simulink subsystem "Rocket_Motor"  (R2020b)
settings: Solver=VariableStepAuto  StartTime=0.0  StopTime=10.0  RelTol=1e-3
undefined symbols (not defined in the file): LocalRestrictions
libraries: fl_lib x27, nesl_utility x18
settings Model: Creator=Edward  LastModifiedBy=Rafal

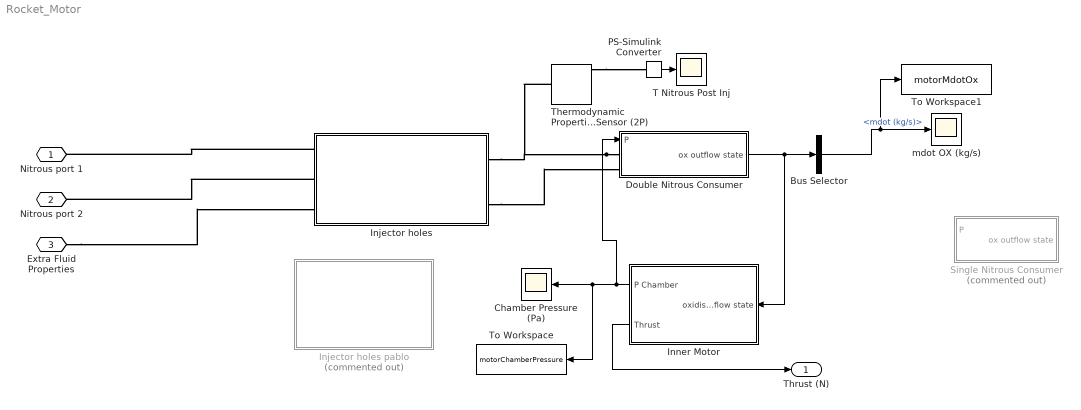
== system Rocket_Motor ==
  Bus Selector : BusSelector  OutputSignals=mdot (kg/s)
  Chamber Pressure (Pa) : Scope
  Double Nitrous Consumer : Subsystem
  Injector holes : Subsystem  Variant=on  VariantControlMode=label  VariantControl=Choice  LabelModeActiveChoice=Omega Modified
  Injector holes pablo : Subsystem  Commented=on
  Inner Motor : Subsystem
      mask Display: image('$imagefile'); % Use "Edit Image" on toolstrip to change.
  PS-Simulink Converter : nesl_utility/PS-Simulink Converter  PhysicalDomain=network_engine_domain  SubClassName=ps_output  LeftPortType=input  RightPortType=output  PseudoPeriodic=off  Frequencies=[]  Unit=inherit  AffineConversion=off
  Single Nitrous Consumer : Subsystem  Commented=on
  T Nitrous Post Inj : Scope
  Thermodynamic Properties Sensor (2P) : fl_lib/Two-Phase Fluid/Sensors/Thermodynamic Properties Sensor (2P)
      settings: SourceProductBaseCode=SS  InternalSimscapePortConfiguration="{\"Bottom\":[],\"Left\":[{\"id\":\"A\",\"label\":\"A\",\"type\":\"foundation.two_phase_fluid.two_phase_fluid\"}],\"Right\":[{\"id\":\"T\",\"label\":\"T\",\"type\":\"output\"},{\"id\":\"H\",\"label\":\"h\",\"type\":\"output\"},{\"id\":\"V\",\"label\":\"v\",\"type\":\"output\"},{\"id\":\"S\",\"label\":\"s\",\"type\":\"output\"}],\"Top\":[]}"
  To Workspace : ToWorkspace  VariableName=motorChamberPressure  SaveFormat=Timeseries  SampleTime=-1
  To Workspace1 : ToWorkspace  VariableName=motorMdotOx  SaveFormat=Timeseries  SampleTime=-1
  mdot OX (kg/s) : Scope
  Nitrous port 1 : PMIOPort  Side=Left
  Nitrous port 2 : PMIOPort  Port=2  Side=Left
  Extra Fluid Properties : PMIOPort  Port=3  Side=Left
  Thrust (N) : Outport
  wires:
  Bus Selector/1 -> mdot OX (kg/s)/1, To Workspace1/1  "<mdot (kg/s)>"
  Inner Motor/1(P Chamber) -> To Workspace/1, Chamber Pressure (Pa)/1, Double Nitrous Consumer/1(P)
  Inner Motor/2(Thrust) -> Thrust (N)/1
  PS-Simulink Converter/1 -> T Nitrous Post Inj/1
  Double Nitrous Consumer/1(ox outflow state) -> Bus Selector/1, Inner Motor/1(oxidiser inflow state)
  connections:
  Double Nitrous Consumer/LConn1 -- Thermodynamic Properties Sensor (2P)/LConn1 -- Injector holes/RConn1
  Thermodynamic Properties Sensor (2P)/RConn1 -- PS-Simulink Converter/LConn1
  Injector holes/LConn1 -- Nitrous port 1/RConn1
  Injector holes/LConn2 -- Nitrous port 2/RConn1
  Injector holes/RConn2 -- Double Nitrous Consumer/LConn2
  Extra Fluid Properties/RConn1 -- Injector holes/LConn3

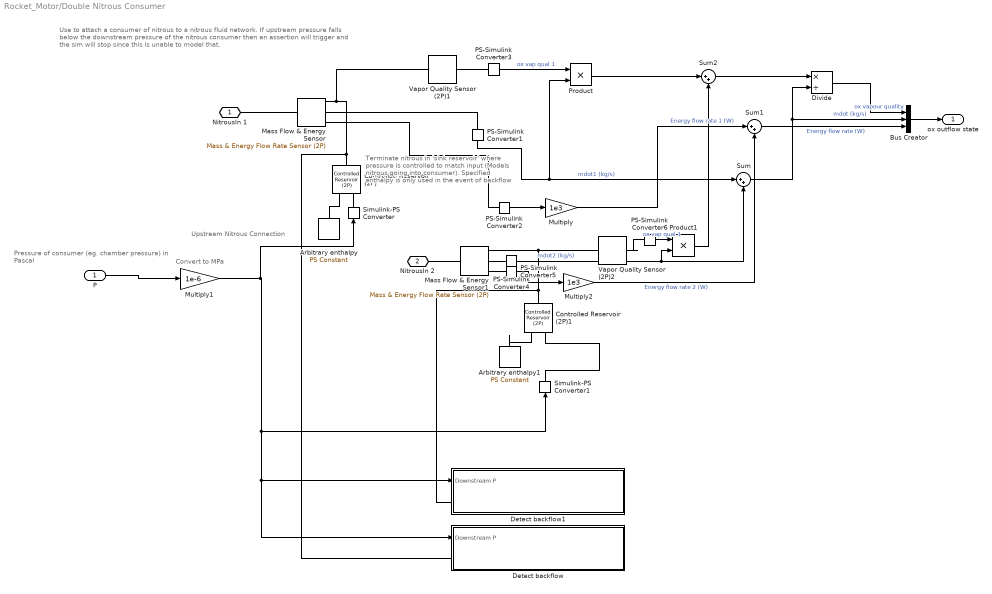
== system Rocket_Motor/Double Nitrous Consumer ==
  note: Pressure of consumer (eg. chamber pressure)
      | in Pascal
  note: Upstream Nitrous Connection
  note: Terminate nitrous in 'sink reservoir'
      | where pressure is controlled to
      | match input (Models nitrous going into
      | consumer). Specified enthalpy is only used
      | in the event of backflow
  note: Convert to MPa
  note: Use to attach a consumer of nitrous to a nitrous fluid network.
      |
      | If upstream pressure falls below the downstream pressure of the nitrous
      | consumer then an assertion will trigger and the sim will stop since
      | this is unable to model that.
  P : Inport
  Arbitrary enthalpy : fl_lib/Physical Signals/Sources/PS Constant  constant=362 kJ/kg
  Arbitrary enthalpy1 : fl_lib/Physical Signals/Sources/PS Constant  constant=362 kJ/kg
  Bus Creator : BusCreator  Inputs=3
  Controlled Reservoir (2P) : fl_lib/Two-Phase Fluid/Elements/Controlled Reservoir (2P)  energy_spec=foundation.enum.enthalpy_internal_energy_spec.enthalpy  area_A=Sim.injector.postInjectorCrossSection m^2
      settings: SourceProductBaseCode=SS  InternalSimscapePortConfiguration="{\"Bottom\":[],\"Left\":[{\"id\":\"A\",\"label\":\"A\",\"type\":\"foundation.two_phase_fluid.two_phase_fluid\"}],\"Right\":[{\"id\":\"H\",\"label\":\"H\",\"type\":\"input\"},{\"id\":\"P\",\"label\":\"P\",\"type\":\"input\"}],\"Top\":[]}"
  Controlled Reservoir (2P)1 : fl_lib/Two-Phase Fluid/Elements/Controlled Reservoir (2P)  energy_spec=foundation.enum.enthalpy_internal_energy_spec.enthalpy  area_A=Sim.injector.postInjectorCrossSection m^2
      settings: SourceProductBaseCode=SS  InternalSimscapePortConfiguration="{\"Bottom\":[],\"Left\":[{\"id\":\"A\",\"label\":\"A\",\"type\":\"foundation.two_phase_fluid.two_phase_fluid\"}],\"Right\":[{\"id\":\"H\",\"label\":\"H\",\"type\":\"input\"},{\"id\":\"P\",\"label\":\"P\",\"type\":\"input\"}],\"Top\":[]}"
  Detect backflow : Subsystem
  Detect backflow1 : Subsystem
  Divide : Product  Inputs=*/
  Mass Flow & Energy Sensor : fl_lib/Two-Phase Fluid/Sensors/Mass & Energy Flow Rate Sensor (2P)
      settings: SourceProductBaseCode=SS  InternalSimscapePortConfiguration="{\"Bottom\":[],\"Left\":[{\"id\":\"A\",\"label\":\"A\",\"type\":\"foundation.two_phase_fluid.two_phase_fluid\"}],\"Right\":[{\"id\":\"B\",\"label\":\"B\",\"type\":\"foundation.two_phase_fluid.two_phase_fluid\"},{\"id\":\"M\",\"label\":\"M\",\"type\":\"output\"},{\"id\":\"PHI\",\"label\":\"Phi\",\"type\":\"output\"}],\"Top\":[]}"
  Mass Flow & Energy Sensor1 : fl_lib/Two-Phase Fluid/Sensors/Mass & Energy Flow Rate Sensor (2P)
      settings: SourceProductBaseCode=SS  InternalSimscapePortConfiguration="{\"Bottom\":[],\"Left\":[{\"id\":\"A\",\"label\":\"A\",\"type\":\"foundation.two_phase_fluid.two_phase_fluid\"}],\"Right\":[{\"id\":\"B\",\"label\":\"B\",\"type\":\"foundation.two_phase_fluid.two_phase_fluid\"},{\"id\":\"M\",\"label\":\"M\",\"type\":\"output\"},{\"id\":\"PHI\",\"label\":\"Phi\",\"type\":\"output\"}],\"Top\":[]}"
  Multiply : Gain  Gain=1e3
  Multiply1 : Gain  Gain=1e-6
  Multiply2 : Gain  Gain=1e3
  PS-Simulink Converter{1..6} (6 alike) : nesl_utility/PS-Simulink Converter  PhysicalDomain=network_engine_domain  SubClassName=ps_output  LeftPortType=input  RightPortType=output  PseudoPeriodic=off  Frequencies=[]  Unit=inherit  AffineConversion=off
  Product : Product
  Product1 : Product
  Simulink-PS Converter : nesl_utility/Simulink-PS Converter  PhysicalDomain=network_engine_domain  SubClassName=ps_input  LeftPortType=input  RightPortType=output  PseudoPeriodic=off  Frequencies=[]  NoiseDistribution=none  NoiseParameters=[]  Unit=1  AffineConversion=off  FilteringAndDerivatives=provide  SimscapeFilterOrder=1  InputFilterTimeConstant=0.001  UdotUserProvided=0
  Simulink-PS Converter1 : nesl_utility/Simulink-PS Converter  PhysicalDomain=network_engine_domain  SubClassName=ps_input  LeftPortType=input  RightPortType=output  PseudoPeriodic=off  Frequencies=[]  NoiseDistribution=none  NoiseParameters=[]  Unit=1  AffineConversion=off  FilteringAndDerivatives=provide  SimscapeFilterOrder=1  InputFilterTimeConstant=0.001  UdotUserProvided=0
  Sum : Sum  Inputs=|++
  Sum1 : Sum  Inputs=|++
  Sum2 : Sum  Inputs=|++
  Vapor Quality Sensor (2P)1 : fl_lib/Two-Phase Fluid/Sensors/Vapor Quality Sensor (2P)  vapor_fraction_spec=foundation.enum.vapor_fraction_spec.quality
      settings: SourceProductBaseCode=SS  InternalSimscapePortConfiguration="{\"Bottom\":[],\"Left\":[{\"id\":\"A\",\"label\":\"A\",\"type\":\"foundation.two_phase_fluid.two_phase_fluid\"}],\"Right\":[{\"id\":\"X\",\"label\":\"X\",\"type\":\"output\"}],\"Top\":[]}"
  Vapor Quality Sensor (2P)2 : fl_lib/Two-Phase Fluid/Sensors/Vapor Quality Sensor (2P)  vapor_fraction_spec=foundation.enum.vapor_fraction_spec.quality
      settings: SourceProductBaseCode=SS  InternalSimscapePortConfiguration="{\"Bottom\":[],\"Left\":[{\"id\":\"A\",\"label\":\"A\",\"type\":\"foundation.two_phase_fluid.two_phase_fluid\"}],\"Right\":[{\"id\":\"X\",\"label\":\"X\",\"type\":\"output\"}],\"Top\":[]}"
  NitrousIn 1 : PMIOPort  Side=Left
  NitrousIn 2 : PMIOPort  Port=2  Side=Left
  ox outflow state : Outport
  wires:
  Divide/1 -> Bus Creator/1  "ox vapour quality"
  Sum2/1 -> Divide/1
  Product/1 -> Sum2/1
  Product1/1 -> Sum2/2
  PS-Simulink Converter6/1 -> Product1/1  "ox vap qual 1"
  PS-Simulink Converter3/1 -> Product/1  "ox vap qual 1"
  Sum1/1 -> Bus Creator/3  "Energy flow rate (W)"
  Sum/1 -> Bus Creator/2, Divide/2  "mdot (kg/s)"
  Multiply2/1 -> Sum1/2  "Energy flow rate 2 (W)"
  PS-Simulink Converter4/1 -> Sum/2, Product1/2  "mdot2 (kg/s)"
  PS-Simulink Converter5/1 -> Multiply2/1
  Bus Creator/1 -> ox outflow state/1
  Multiply1/1 -> Simulink-PS Converter/1, Detect backflow/1(Downstream P), Detect backflow1/1(Downstream P), Simulink-PS Converter1/1
  Multiply/1 -> Sum1/1  "Energy flow rate 1 (W)"
  PS-Simulink Converter2/1 -> Multiply/1
  P/1 -> Multiply1/1
  PS-Simulink Converter1/1 -> Sum/1, Product/2  "mdot1 (kg/s)"
  connections:
  Simulink-PS Converter1/RConn1 -- Controlled Reservoir (2P)1/RConn2
  Arbitrary enthalpy1/RConn1 -- Controlled Reservoir (2P)1/RConn1
  Vapor Quality Sensor (2P)2/RConn1 -- PS-Simulink Converter6/LConn1
  PS-Simulink Converter5/LConn1 -- Mass Flow & Energy Sensor1/RConn3
  PS-Simulink Converter4/LConn1 -- Mass Flow & Energy Sensor1/RConn2
  Mass Flow & Energy Sensor1/RConn1 -- Vapor Quality Sensor (2P)2/LConn1 -- Controlled Reservoir (2P)1/LConn1 -- Detect backflow1/LConn1
  Mass Flow & Energy Sensor1/LConn1 -- NitrousIn 2/RConn1
  Detect backflow/LConn1 -- Controlled Reservoir (2P)/LConn1 -- Vapor Quality Sensor (2P)1/LConn1 -- Mass Flow & Energy Sensor/RConn1
  Vapor Quality Sensor (2P)1/RConn1 -- PS-Simulink Converter3/LConn1
  Mass Flow & Energy Sensor/LConn1 -- NitrousIn 1/RConn1
  Mass Flow & Energy Sensor/RConn3 -- PS-Simulink Converter2/LConn1
  Mass Flow & Energy Sensor/RConn2 -- PS-Simulink Converter1/LConn1
  Arbitrary enthalpy/RConn1 -- Controlled Reservoir (2P)/RConn1
  Simulink-PS Converter/RConn1 -- Controlled Reservoir (2P)/RConn2

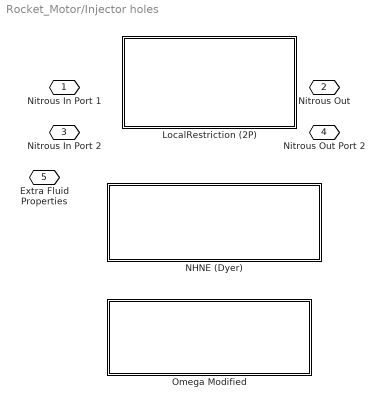
== system Rocket_Motor/Injector holes ==
  LocalRestriction (2P) : Subsystem  VariantControl=LocalRestrictions (2P)  ReferencedSubsystem=Injector  dischargeCoeff=0.64
  NHNE (Dyer) : Subsystem  VariantControl=NHNE (Dyer)  ReferencedSubsystem=InjectorNHNE  dischargeCoeff=0.64  numHolesPort1=Sim.injector.numHolesPort1  numHolesPort2=Sim.injector.numHolesPort2  holeAreaPort1=Sim.injector.singleHoleAPort1  holeAreaPort2=Sim.injector.singleHoleAPort2
  Omega Modified : Subsystem  VariantControl=Omega Modified  ReferencedSubsystem=InjectorOmega  CdOmegaLow=0.85  CdOmegaHigh=0.73  KExcessPressureDrop=2.28  numHolesPort1=Sim.injector.numHolesPort1  numHolesPort2=Sim.injector.numHolesPort2  holeDiamPort1=Sim.injector.singleHoleDiamPort1  holeDiamPort2=Sim.injector.singleHoleDiamPort2  LInjector=Sim.injector.injectorDepth
  Nitrous In Port 1 : PMIOPort  Side=Left
  Nitrous Out : PMIOPort  Port=2  Side=Right
  Nitrous In Port 2 : PMIOPort  Port=3  Side=Left
  Nitrous Out Port 2 : PMIOPort  Port=4  Side=Right
  Extra Fluid Properties : PMIOPort  Port=5  Side=Left

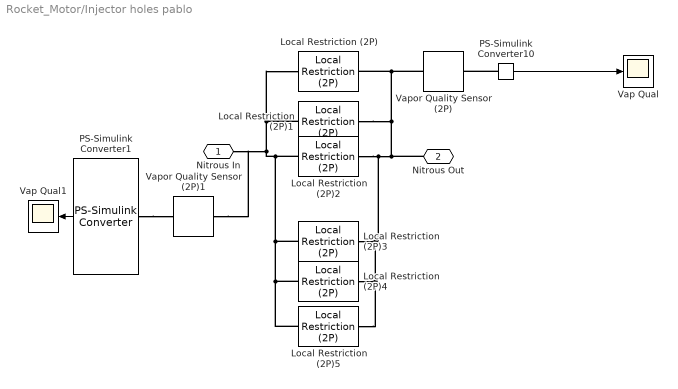
== system Rocket_Motor/Injector holes pablo ==
  Local Restriction (2P) : fl_lib/Two-Phase Fluid/Elements/Local Restriction (2P)  restriction_area=9.50e-7 m^2  area=sim.preInjectorPipe.crossSection m^2  Cd=0.64  B_lam=0.999
      settings: SourceProductBaseCode=SS  InternalSimscapePortConfiguration="{\"Bottom\":[],\"Left\":[{\"id\":\"A\",\"label\":\"A\",\"type\":\"foundation.two_phase_fluid.two_phase_fluid\"}],\"Right\":[{\"id\":\"B\",\"label\":\"B\",\"type\":\"foundation.two_phase_fluid.two_phase_fluid\"}],\"Top\":[]}"
  Local Restriction (2P)1 : fl_lib/Two-Phase Fluid/Elements/Local Restriction (2P)  restriction_area=9.50e-7 m^2  area=sim.preInjectorPipe.crossSection m^2  Cd=0.64  B_lam=0.999
      settings: SourceProductBaseCode=SS  InternalSimscapePortConfiguration="{\"Bottom\":[],\"Left\":[{\"id\":\"A\",\"label\":\"A\",\"type\":\"foundation.two_phase_fluid.two_phase_fluid\"}],\"Right\":[{\"id\":\"B\",\"label\":\"B\",\"type\":\"foundation.two_phase_fluid.two_phase_fluid\"}],\"Top\":[]}"
  Local Restriction (2P)2 : fl_lib/Two-Phase Fluid/Elements/Local Restriction (2P)  restriction_area=9.50e-7 m^2  area=sim.preInjectorPipe.crossSection m^2  Cd=0.64  B_lam=0.999
      settings: SourceProductBaseCode=SS  InternalSimscapePortConfiguration="{\"Bottom\":[],\"Left\":[{\"id\":\"A\",\"label\":\"A\",\"type\":\"foundation.two_phase_fluid.two_phase_fluid\"}],\"Right\":[{\"id\":\"B\",\"label\":\"B\",\"type\":\"foundation.two_phase_fluid.two_phase_fluid\"}],\"Top\":[]}"
  Local Restriction (2P)3 : fl_lib/Two-Phase Fluid/Elements/Local Restriction (2P)  restriction_area=4.07e-7 m^2  area=sim.preInjectorPipe.crossSection m^2  Cd=0.64  B_lam=0.999
      settings: SourceProductBaseCode=SS  InternalSimscapePortConfiguration="{\"Bottom\":[],\"Left\":[{\"id\":\"A\",\"label\":\"A\",\"type\":\"foundation.two_phase_fluid.two_phase_fluid\"}],\"Right\":[{\"id\":\"B\",\"label\":\"B\",\"type\":\"foundation.two_phase_fluid.two_phase_fluid\"}],\"Top\":[]}"
  Local Restriction (2P)4 : fl_lib/Two-Phase Fluid/Elements/Local Restriction (2P)  restriction_area=4.07e-7 m^2  area=sim.preInjectorPipe.crossSection m^2  Cd=0.64  B_lam=0.999
      settings: SourceProductBaseCode=SS  InternalSimscapePortConfiguration="{\"Bottom\":[],\"Left\":[{\"id\":\"A\",\"label\":\"A\",\"type\":\"foundation.two_phase_fluid.two_phase_fluid\"}],\"Right\":[{\"id\":\"B\",\"label\":\"B\",\"type\":\"foundation.two_phase_fluid.two_phase_fluid\"}],\"Top\":[]}"
  Local Restriction (2P)5 : fl_lib/Two-Phase Fluid/Elements/Local Restriction (2P)  restriction_area=4.07e-7 m^2  area=sim.preInjectorPipe.crossSection m^2  Cd=0.64  B_lam=0.999
      settings: SourceProductBaseCode=SS  InternalSimscapePortConfiguration="{\"Bottom\":[],\"Left\":[{\"id\":\"A\",\"label\":\"A\",\"type\":\"foundation.two_phase_fluid.two_phase_fluid\"}],\"Right\":[{\"id\":\"B\",\"label\":\"B\",\"type\":\"foundation.two_phase_fluid.two_phase_fluid\"}],\"Top\":[]}"
  PS-Simulink Converter1 : nesl_utility/PS-Simulink Converter  PhysicalDomain=network_engine_domain  SubClassName=ps_output  LeftPortType=input  RightPortType=output  PseudoPeriodic=off  Frequencies=[]  Unit=inherit  AffineConversion=off
  PS-Simulink Converter10 : nesl_utility/PS-Simulink Converter  PhysicalDomain=network_engine_domain  SubClassName=ps_output  LeftPortType=input  RightPortType=output  PseudoPeriodic=off  Frequencies=[]  Unit=inherit  AffineConversion=off
  Vap Qual : Scope
  Vap Qual1 : Scope
  Vapor Quality Sensor (2P) : fl_lib/Two-Phase Fluid/Sensors/Vapor Quality Sensor (2P)  vapor_fraction_spec=foundation.enum.vapor_fraction_spec.quality
      settings: SourceProductBaseCode=SS  InternalSimscapePortConfiguration="{\"Bottom\":[],\"Left\":[{\"id\":\"A\",\"label\":\"A\",\"type\":\"foundation.two_phase_fluid.two_phase_fluid\"}],\"Right\":[{\"id\":\"X\",\"label\":\"X\",\"type\":\"output\"}],\"Top\":[]}"
  Vapor Quality Sensor (2P)1 : fl_lib/Two-Phase Fluid/Sensors/Vapor Quality Sensor (2P)  vapor_fraction_spec=foundation.enum.vapor_fraction_spec.quality
      settings: SourceProductBaseCode=SS  InternalSimscapePortConfiguration="{\"Bottom\":[],\"Left\":[{\"id\":\"A\",\"label\":\"A\",\"type\":\"foundation.two_phase_fluid.two_phase_fluid\"}],\"Right\":[{\"id\":\"X\",\"label\":\"X\",\"type\":\"output\"}],\"Top\":[]}"
  Nitrous In : PMIOPort  Side=Left
  Nitrous Out : PMIOPort  Port=2  Side=Right
  wires:
  PS-Simulink Converter1/1 -> Vap Qual1/1
  PS-Simulink Converter10/1 -> Vap Qual/1
  connections:
  PS-Simulink Converter1/LConn1 -- Vapor Quality Sensor (2P)1/RConn1
  PS-Simulink Converter10/LConn1 -- Vapor Quality Sensor (2P)/RConn1
  Local Restriction (2P)4/LConn1 -- Local Restriction (2P)5/LConn1 -- Local Restriction (2P)3/LConn1 -- Local Restriction (2P)2/LConn1 -- Vapor Quality Sensor (2P)1/LConn1 -- Nitrous In/RConn1 -- Local Restriction (2P)/LConn1 -- Local Restriction (2P)1/LConn1
  Local Restriction (2P)5/RConn1 -- Local Restriction (2P)4/RConn1 -- Local Restriction (2P)3/RConn1 -- Local Restriction (2P)2/RConn1 -- Local Restriction (2P)/RConn1 -- Vapor Quality Sensor (2P)/LConn1 -- Local Restriction (2P)1/RConn1 -- Nitrous Out/RConn1

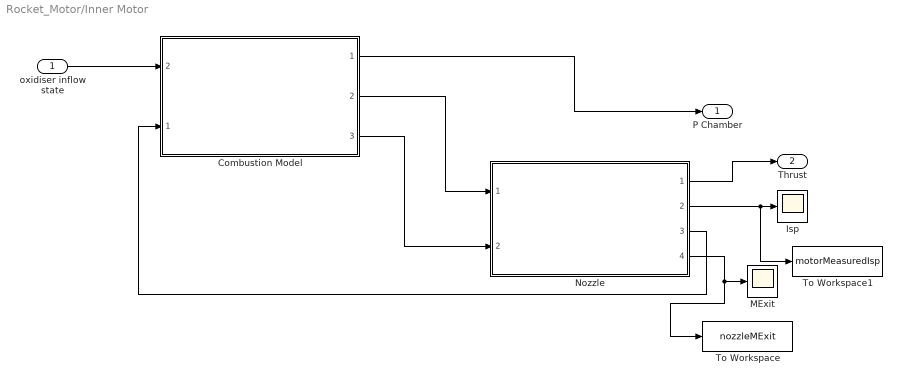
== system Rocket_Motor/Inner Motor ==
  oxidiser inflow state : Inport
  Combustion Model : Subsystem  ReferencedSubsystem=Combustion_Model  useOxidiserFluxOnlyRegRateEquation=Sim.combustionChamber.useOxFluxRegRateEquation
      settings: PortSchema="{\"entries\":[{\"content\":{\"sides\":[{\"content\":{\"connectorIds\":[\"In2\",\"In1\"]},\"type\":\"ConnectorPlacement.EquallySpacedRectSide\",\"uuid\":\"69910484-f410-42d1-a1e3-8cbed6938d6d\"},{\"content\":{\"connectorIds\":[\"Out1\",\"Out2\",\"Out3\"],\"side\":\"RIGHT\"},\"type\":\"ConnectorPlacement.EquallySpacedRectSide\",\"uuid\":\"6ec29124-1872-48dc-b93d-2641f1613bb4\"},{\"content\":{\"connectorIds\":[],\"side\":\"TOP\"},\"type\":\"ConnectorPlacement.EquallySpacedRectSide\",\"uuid\":\"79a0fe1d-0cb1-4f18-8d79-fe4459103554\"},{\"content\":{\"connectorIds\":[],\"side\":\"HIDDEN\"},\"type\":\"ConnectorPlacement.EquallySpacedRectSide\",\"uuid\":\"d348ca01-66ec-489a-a521-91dc415e5dea\"}]},\"type\":\"ConnectorPlacement.EquallySpacedConnector\",\"uuid\":\"f28a91d1-95ea-44a7-b053-f5f076a7433e\"}],\"packageUris\":[\"http://schema.mathworks.com/mf0/Connector/R2020b\"],\"version\":\"1.0\"}"
  Isp : Scope
  MExit : Scope
  Nozzle : Subsystem  ReferencedSubsystem=Nozzle
  To Workspace : ToWorkspace  VariableName=nozzleMExit  SaveFormat=Timeseries  SampleTime=-1
  To Workspace1 : ToWorkspace  VariableName=motorMeasuredIsp  SaveFormat=Timeseries  SampleTime=-1
  P Chamber : Outport
  Thrust : Outport  Port=2
  wires:
  Combustion Model/3 -> Nozzle/2
  oxidiser inflow state/1 -> Combustion Model/2
  Nozzle/3 -> Combustion Model/1
  Nozzle/4 -> MExit/1, To Workspace/1
  Nozzle/2 -> Isp/1, To Workspace1/1
  Nozzle/1 -> Thrust/1
  Combustion Model/2 -> Nozzle/1
  Combustion Model/1 -> P Chamber/1

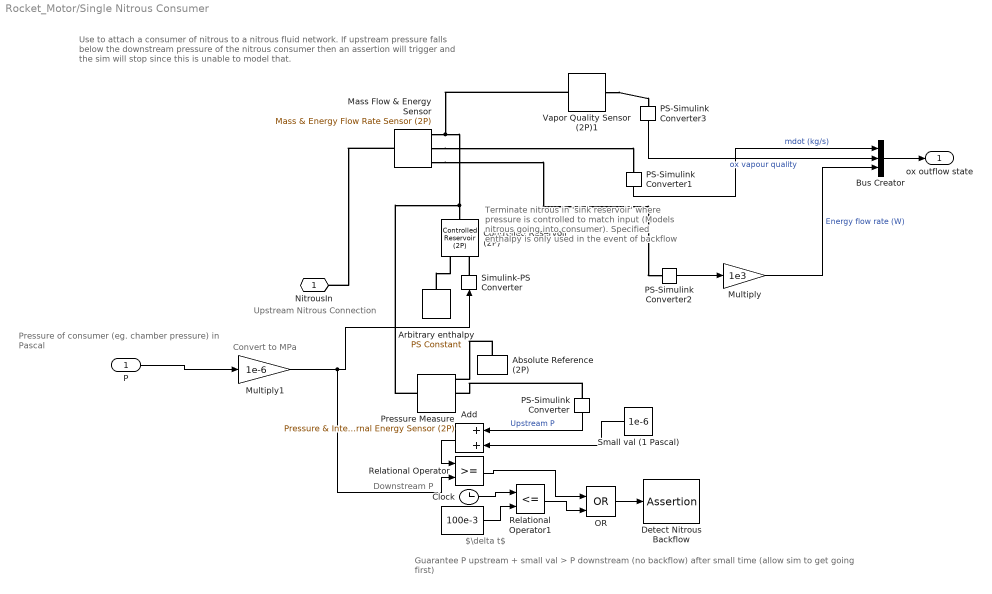
== system Rocket_Motor/Single Nitrous Consumer ==
  note: Pressure of consumer (eg. chamber pressure)
      | in Pascal
  note: Upstream Nitrous Connection
  note: Downstream P
  note: Guarantee P upstream + small val > P downstream (no backflow) after small time (allow sim to get going first)
  note: Terminate nitrous in 'sink reservoir'
      | where pressure is controlled to
      | match input (Models nitrous going into
      | consumer). Specified enthalpy is only used
      | in the event of backflow
  note: Convert to MPa
  note: Use to attach a consumer of nitrous to a nitrous fluid network.
      |
      | If upstream pressure falls below the downstream pressure of the nitrous
      | consumer then an assertion will trigger and the sim will stop since
      | this is unable to model that.
  note: $\delta t$
  P : Inport
  " " : Constant  Value=100e-3
  Absolute Reference (2P) : fl_lib/Two-Phase Fluid/Elements/Absolute Reference (2P)
      settings: SourceProductBaseCode=SS
  Add : Sum
  Arbitrary enthalpy : fl_lib/Physical Signals/Sources/PS Constant  constant=362 kJ/kg
  Bus Creator : BusCreator  Inputs=3
  Clock : Clock
  Controlled Reservoir (2P) : fl_lib/Two-Phase Fluid/Elements/Controlled Reservoir (2P)  energy_spec=foundation.enum.enthalpy_internal_energy_spec.enthalpy  area_A=Sim.injector.postInjectorCrossSection m^2
      settings: SourceProductBaseCode=SS  InternalSimscapePortConfiguration="{\"Bottom\":[],\"Left\":[{\"id\":\"A\",\"label\":\"A\",\"type\":\"foundation.two_phase_fluid.two_phase_fluid\"}],\"Right\":[{\"id\":\"H\",\"label\":\"H\",\"type\":\"input\"},{\"id\":\"P\",\"label\":\"P\",\"type\":\"input\"}],\"Top\":[]}"
  Detect Nitrous Backflow : Assertion
  Mass Flow & Energy Sensor : fl_lib/Two-Phase Fluid/Sensors/Mass & Energy Flow Rate Sensor (2P)
      settings: SourceProductBaseCode=SS  InternalSimscapePortConfiguration="{\"Bottom\":[],\"Left\":[{\"id\":\"A\",\"label\":\"A\",\"type\":\"foundation.two_phase_fluid.two_phase_fluid\"}],\"Right\":[{\"id\":\"B\",\"label\":\"B\",\"type\":\"foundation.two_phase_fluid.two_phase_fluid\"},{\"id\":\"M\",\"label\":\"M\",\"type\":\"output\"},{\"id\":\"PHI\",\"label\":\"Phi\",\"type\":\"output\"}],\"Top\":[]}"
  Multiply : Gain  Gain=1e3
  Multiply1 : Gain  Gain=1e-6
  OR : Logic  Operator=OR  IconShape=distinctive  AllPortsSameDT=off  OutDataTypeStr=boolean
  PS-Simulink Converter{,1..3} (4 alike) : nesl_utility/PS-Simulink Converter  PhysicalDomain=network_engine_domain  SubClassName=ps_output  LeftPortType=input  RightPortType=output  PseudoPeriodic=off  Frequencies=[]  Unit=inherit  AffineConversion=off
  Pressure Measure : fl_lib/Two-Phase Fluid/Sensors/Pressure & Internal Energy Sensor (2P)
      settings: SourceProductBaseCode=SS  InternalSimscapePortConfiguration="{\"Bottom\":[],\"Left\":[{\"id\":\"A\",\"label\":\"A\",\"type\":\"foundation.two_phase_fluid.two_phase_fluid\"}],\"Right\":[{\"id\":\"B\",\"label\":\"B\",\"type\":\"foundation.two_phase_fluid.two_phase_fluid\"},{\"id\":\"P\",\"label\":\"P\",\"type\":\"output\"},{\"id\":\"U\",\"label\":\"U\",\"type\":\"output\"}],\"Top\":[]}"
  Relational Operator : RelationalOperator  OutDataTypeStr=boolean  RndMeth=Simplest
  Relational Operator1 : RelationalOperator  Operator=<=  OutDataTypeStr=boolean  RndMeth=Simplest
  Simulink-PS Converter : nesl_utility/Simulink-PS Converter  PhysicalDomain=network_engine_domain  SubClassName=ps_input  LeftPortType=input  RightPortType=output  PseudoPeriodic=off  Frequencies=[]  NoiseDistribution=none  NoiseParameters=[]  Unit=1  AffineConversion=off  FilteringAndDerivatives=provide  SimscapeFilterOrder=1  InputFilterTimeConstant=0.001  UdotUserProvided=0
  Small val (1 Pascal) : Constant  Value=1e-6
  Vapor Quality Sensor (2P)1 : fl_lib/Two-Phase Fluid/Sensors/Vapor Quality Sensor (2P)  vapor_fraction_spec=foundation.enum.vapor_fraction_spec.quality
      settings: SourceProductBaseCode=SS  InternalSimscapePortConfiguration="{\"Bottom\":[],\"Left\":[{\"id\":\"A\",\"label\":\"A\",\"type\":\"foundation.two_phase_fluid.two_phase_fluid\"}],\"Right\":[{\"id\":\"X\",\"label\":\"X\",\"type\":\"output\"}],\"Top\":[]}"
  NitrousIn : PMIOPort  Side=Left
  ox outflow state : Outport
  wires:
  Bus Creator/1 -> ox outflow state/1
  OR/1 -> Detect Nitrous Backflow/1
  Relational Operator1/1 -> OR/2
  " "/1 -> Relational Operator1/2
  Clock/1 -> Relational Operator1/1
  Small val (1 Pascal)/1 -> Add/2
  Add/1 -> Relational Operator/1
  PS-Simulink Converter/1 -> Add/1  "Upstream P"
  PS-Simulink Converter3/1 -> Bus Creator/2  "ox vapour quality"
  Multiply1/1 -> Simulink-PS Converter/1, Relational Operator/2
  Multiply/1 -> Bus Creator/3  "Energy flow rate (W)"
  PS-Simulink Converter2/1 -> Multiply/1
  P/1 -> Multiply1/1
  PS-Simulink Converter1/1 -> Bus Creator/1  "mdot (kg/s)"
  Relational Operator/1 -> OR/1
  connections:
  Vapor Quality Sensor (2P)1/RConn1 -- PS-Simulink Converter3/LConn1
  Mass Flow & Energy Sensor/LConn1 -- NitrousIn/RConn1
  Mass Flow & Energy Sensor/RConn3 -- PS-Simulink Converter2/LConn1
  Mass Flow & Energy Sensor/RConn2 -- PS-Simulink Converter1/LConn1
  PS-Simulink Converter/LConn1 -- Pressure Measure/RConn2
  Absolute Reference (2P)/LConn1 -- Pressure Measure/RConn1
  Controlled Reservoir (2P)/LConn1 -- Pressure Measure/LConn1 -- Vapor Quality Sensor (2P)1/LConn1 -- Mass Flow & Energy Sensor/RConn1
  Arbitrary enthalpy/RConn1 -- Controlled Reservoir (2P)/RConn1
  Simulink-PS Converter/RConn1 -- Controlled Reservoir (2P)/RConn2

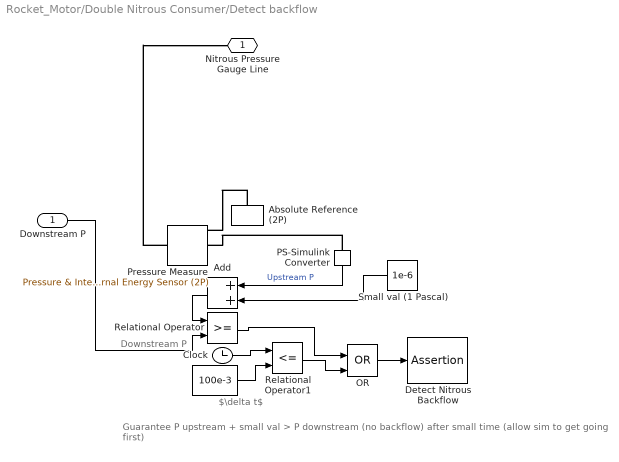
== system Rocket_Motor/Double Nitrous Consumer/Detect backflow ==
  note: Guarantee P upstream + small val > P downstream (no backflow) after small time (allow sim to get going first)
  note: Downstream P
  note: $\delta t$
  Downstream P : Inport
  " " : Constant  Value=100e-3
  Absolute Reference (2P) : fl_lib/Two-Phase Fluid/Elements/Absolute Reference (2P)
      settings: SourceProductBaseCode=SS
  Add : Sum
  Clock : Clock
  Detect Nitrous Backflow : Assertion
  OR : Logic  Operator=OR  IconShape=distinctive  AllPortsSameDT=off  OutDataTypeStr=boolean
  PS-Simulink Converter : nesl_utility/PS-Simulink Converter  PhysicalDomain=network_engine_domain  SubClassName=ps_output  LeftPortType=input  RightPortType=output  PseudoPeriodic=off  Frequencies=[]  Unit=inherit  AffineConversion=off
  Pressure Measure : fl_lib/Two-Phase Fluid/Sensors/Pressure & Internal Energy Sensor (2P)
      settings: SourceProductBaseCode=SS  InternalSimscapePortConfiguration="{\"Bottom\":[],\"Left\":[{\"id\":\"A\",\"label\":\"A\",\"type\":\"foundation.two_phase_fluid.two_phase_fluid\"}],\"Right\":[{\"id\":\"B\",\"label\":\"B\",\"type\":\"foundation.two_phase_fluid.two_phase_fluid\"},{\"id\":\"P\",\"label\":\"P\",\"type\":\"output\"},{\"id\":\"U\",\"label\":\"U\",\"type\":\"output\"}],\"Top\":[]}"
  Relational Operator : RelationalOperator  OutDataTypeStr=boolean  RndMeth=Simplest
  Relational Operator1 : RelationalOperator  Operator=<=  OutDataTypeStr=boolean  RndMeth=Simplest
  Small val (1 Pascal) : Constant  Value=1e-6
  Nitrous Pressure Gauge Line : PMIOPort  Side=Left
  wires:
  Downstream P/1 -> Relational Operator/2
  Small val (1 Pascal)/1 -> Add/2
  OR/1 -> Detect Nitrous Backflow/1
  PS-Simulink Converter/1 -> Add/1  "Upstream P"
  Relational Operator/1 -> OR/1
  " "/1 -> Relational Operator1/2
  Relational Operator1/1 -> OR/2
  Clock/1 -> Relational Operator1/1
  Add/1 -> Relational Operator/1
  connections:
  Pressure Measure/LConn1 -- Nitrous Pressure Gauge Line/RConn1
  Absolute Reference (2P)/LConn1 -- Pressure Measure/RConn1
  PS-Simulink Converter/LConn1 -- Pressure Measure/RConn2

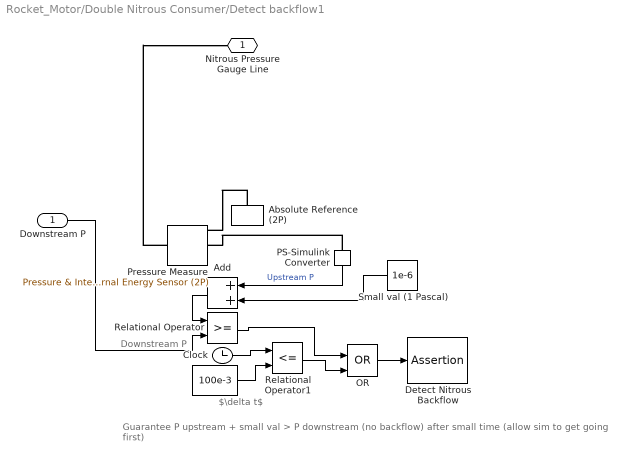
== system Rocket_Motor/Double Nitrous Consumer/Detect backflow1 ==
  note: Guarantee P upstream + small val > P downstream (no backflow) after small time (allow sim to get going first)
  note: Downstream P
  note: $\delta t$
  Downstream P : Inport
  " " : Constant  Value=100e-3
  Absolute Reference (2P) : fl_lib/Two-Phase Fluid/Elements/Absolute Reference (2P)
      settings: SourceProductBaseCode=SS
  Add : Sum
  Clock : Clock
  Detect Nitrous Backflow : Assertion
  OR : Logic  Operator=OR  IconShape=distinctive  AllPortsSameDT=off  OutDataTypeStr=boolean
  PS-Simulink Converter : nesl_utility/PS-Simulink Converter  PhysicalDomain=network_engine_domain  SubClassName=ps_output  LeftPortType=input  RightPortType=output  PseudoPeriodic=off  Frequencies=[]  Unit=inherit  AffineConversion=off
  Pressure Measure : fl_lib/Two-Phase Fluid/Sensors/Pressure & Internal Energy Sensor (2P)
      settings: SourceProductBaseCode=SS  InternalSimscapePortConfiguration="{\"Bottom\":[],\"Left\":[{\"id\":\"A\",\"label\":\"A\",\"type\":\"foundation.two_phase_fluid.two_phase_fluid\"}],\"Right\":[{\"id\":\"B\",\"label\":\"B\",\"type\":\"foundation.two_phase_fluid.two_phase_fluid\"},{\"id\":\"P\",\"label\":\"P\",\"type\":\"output\"},{\"id\":\"U\",\"label\":\"U\",\"type\":\"output\"}],\"Top\":[]}"
  Relational Operator : RelationalOperator  OutDataTypeStr=boolean  RndMeth=Simplest
  Relational Operator1 : RelationalOperator  Operator=<=  OutDataTypeStr=boolean  RndMeth=Simplest
  Small val (1 Pascal) : Constant  Value=1e-6
  Nitrous Pressure Gauge Line : PMIOPort  Side=Left
  wires:
  Downstream P/1 -> Relational Operator/2
  Small val (1 Pascal)/1 -> Add/2
  OR/1 -> Detect Nitrous Backflow/1
  PS-Simulink Converter/1 -> Add/1  "Upstream P"
  Relational Operator/1 -> OR/1
  " "/1 -> Relational Operator1/2
  Relational Operator1/1 -> OR/2
  Clock/1 -> Relational Operator1/1
  Add/1 -> Relational Operator/1
  connections:
  Pressure Measure/LConn1 -- Nitrous Pressure Gauge Line/RConn1
  Absolute Reference (2P)/LConn1 -- Pressure Measure/RConn1
  PS-Simulink Converter/LConn1 -- Pressure Measure/RConn2
